simulink model "hybrid-grid-agc-simulink"  (R2025a)
settings: Solver=VariableStepAuto  StartTime=0.0  StopTime=4  RelTol=1e-3
libraries: spsSeriesRLCBranchLib x2, spsThreePhaseVIMeasurementLib x2, spsControlledVoltageSourceLib x1, spsGroundLib x1, spsPLL3phLib x1, eePwmGeneratorTwoLevel x1, spsSimplifiedSynchronousMachineSIUnitsLib x1, spsSteamTurbineandGovernorLib x1, spsThreePhaseParallelRLCLoadLib x1, spsThreePhaseSourceLib x1, spsUniversalBridgeLib x1, spsVoltageMeasurementLib x1
settings Model: Creator=saranshagrawal  LastModifiedBy=saranshagrawal

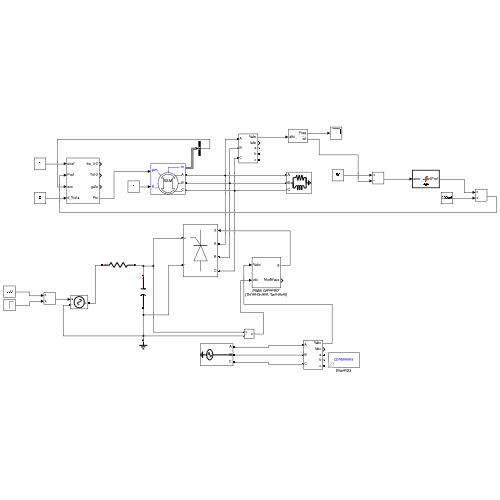
[thumbnail: Simulink's stored preview of the top-level diagram]
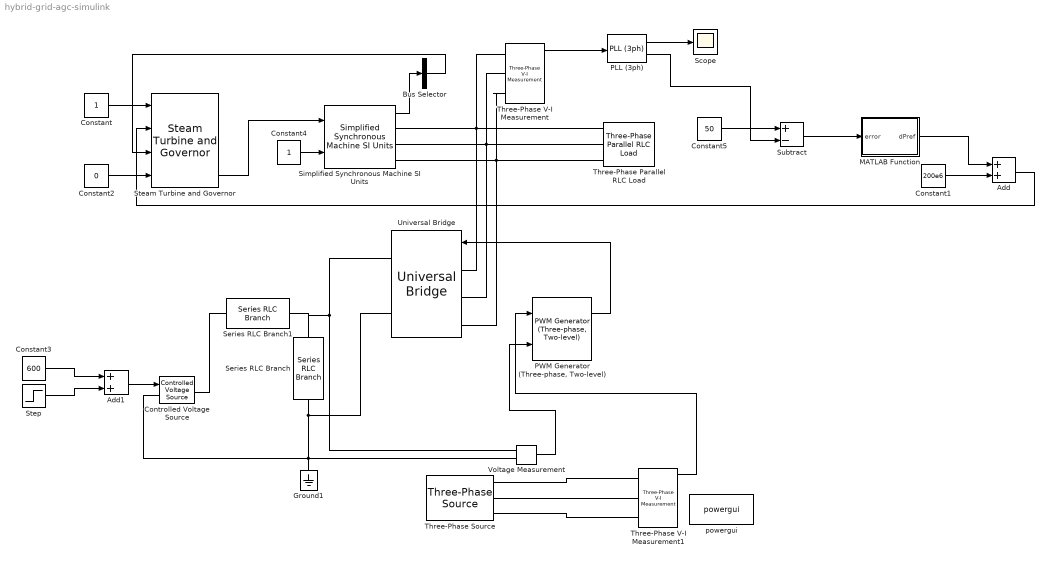
== system hybrid-grid-agc-simulink ==
  Add : Sum
  Add1 : Sum
  Bus Selector : BusSelector  OutputSignals=Rotor speed wm (rad/s)  OutputAsBus=on
  Constant : Constant
  Constant1 : Constant  Value=200e6
  Constant2 : Constant  Value=0
  Constant3 : Constant  Value=600
  Constant4 : Constant
  Constant5 : Constant  Value=50
  Controlled Voltage Source : spsControlledVoltageSourceLib/Controlled Voltage Source  Initialize=on  Source_Type=AC  Amplitude=0  Phase=0  Frequency=0  Measurements=None
  Ground1 : spsGroundLib/Ground  LConnTagsString=a
  MATLAB Function : MATLAB Function  TreatAsAtomicUnit=on
  PLL (3ph) : spsPLL3phLib/PLL (3ph)  Fmin=45  Par_Init=[0, 50]  ParK=[180, 3200, 1]  TcD=1e-4  MaxRateChangeFreq=12  FilterCutOffFreq=25  Ts=0  AGC=on
  "PWM Generator (Three-phase, Two-level)" : eePwmGeneratorTwoLevel/PWM Generator (Three-phase, Two-level)  PWMMode=Continuous PWM (CPWM)  CPWMMode=SPWM: sinusoidal PWM  DPWMMode=60 DPWM: 60 degree discontinuous PWM  fsw=1e3  Ts=5e-5
      settings: LibrarySourceBlock=|
      | ee_sl_lib/Pulse Width
      | Modulation/PWM Generator
      | (Three-phase, Two-level)
  Scope : Scope
      settings: ActiveDisplayYMinimum=49.969171432706709  ActiveDisplayYMaximum=50.039963228671333
  Series RLC Branch : spsSeriesRLCBranchLib/Series RLC Branch  LConnTagsString=__new0  RConnTagsString=__new0  BranchType=C  Resistance=1  Inductance=1e-3  SetiL0=off  InitialCurrent=0  Capacitance=1000e-6  Setx0=off  InitialVoltage=0  Measurements=None
  Series RLC Branch1 : spsSeriesRLCBranchLib/Series RLC Branch  LConnTagsString=__new0  RConnTagsString=__new0  BranchType=R  Resistance=1  Inductance=1e-3  SetiL0=off  InitialCurrent=0  Capacitance=1e-6  Setx0=off  InitialVoltage=0  Measurements=None
  Simplified Synchronous Machine SI Units : spsSimplifiedSynchronousMachineSIUnitsLib/Simplified Synchronous Machine SI Units  ConnectionType=3-wire Y  MechanicalLoad=Mechanical power Pm  MeasurementBus=off  NominalParameters=[187e6 13800 50]  Mechanical=[3.895e6 0 20]  InternalRL="[0.0204  0.8104e-3]"  InitialConditions="[ 0,0   0,0,0   0,0,0 ]"  IterativeDiscreteModel=Trapezoidal non iterative  TsBlock=-1  TsPowergui=0  LoadFlowParameters=[1,0,0,0,0]  Units=1  BusType=PV  Pref=0  Qref=0  Qmin=-inf  Qmax=+inf  PLF=0  QLF=0
      settings: LibrarySourceBlock=|
      | sps_lib/Electrical Machines/Simplified Synchronous
      | Machine SI Units
  Steam Turbine and Governor : spsSteamTurbineandGovernorLib/Steam Turbine and Governor  gentype=Tandem-compound (multi-mass)  reg1="[ 1  0.05    0 ]"  reg2="[ 0.001  0.15 ]"  reg3="[ -0.1  0.1  0  4.496]"  N=3000  turb1="[ 0  10   3.3   0.5   ]"  turb2="[ 0.5   0.5   0  0 ]"  HA="[  1.5498   0.24894  0  0 ]"  KA="[  83.47  42.702  0  0 ]"  DA=[2.4832 0.4 0 0]  ini1=250.35/555  ini2=[0 -120]
      settings: LibrarySourceBlock=|
      | sps_lib/Electrical Machines/Synchronous Machine Control/Steam Turbine
      | and Governor
  Step : Step  Time=2  After=500  SampleTime=0
  Subtract : Sum  Inputs=+-
  Three-Phase Parallel RLC Load : spsThreePhaseParallelRLCLoadLib/Three-Phase Parallel RLC Load  LConnTagsString=A|B|C  Configuration=Y (grounded)  NominalVoltage=1000  Vabc=[1e3 1e3 1e3]  Vabcp=[1e3 1e3 1e3]  NominalFrequency=50  UnbalancedPower=off  ActivePower=40e6  InductivePower=10e6  CapacitivePower=0  Pabc=[10e3 9e3 11e3]  QLabc=[100 90 110]  QCabc=[100 90 110]  Pabcp=[10e3 9e3 11e3]  QLabcp=[100 90 110]  QCabcp=[100 90 110]  Measurements=None  LoadType=constant Z
  Three-Phase V-I Measurement : spsThreePhaseVIMeasurementLib/Three-Phase V-I Measurement  VoltageMeasurement=phase-to-ground  SetLabelV=off  LabelV=Vabc  Vpu=off  VpuLL=off  CurrentMeasurement=yes  SetLabelI=off  LabelI=Iabc  Ipu=off  Pbase=100e6  Vbase=500e3  OutputType=Complex  PhasorSimulation=off  PSBequivalent=0
  Three-Phase V-I Measurement1 : spsThreePhaseVIMeasurementLib/Three-Phase V-I Measurement  VoltageMeasurement=phase-to-ground  SetLabelV=off  LabelV=Vabc  Vpu=off  VpuLL=off  CurrentMeasurement=yes  SetLabelI=off  LabelI=Iabc  Ipu=off  Pbase=100e6  Vbase=500e3  OutputType=Complex  PhasorSimulation=off  PSBequivalent=0
  Three-Phase Source : spsThreePhaseSourceLib/Three-Phase Source  InternalConnection=Yg  VoltagePhases=off  Voltage=1  PhaseAngle=0  Voltage_phases=[25e3 25e3 25e3]/sqrt(3)  PhaseAngles_phases=[0 -120 +120]  Frequency=50  NonIdealSource=on  SpecifyImpedance=off  Resistance=0  Inductance=0  ShortCircuitLevel=100e6  BaseVoltage=1  XRratio=7  BusType=swing  Pref=10e3  Qref=0  Prefabc=[10e3, 10e3, 10e3]  Qrefabc=[0, 0, 0]  Qmin=-inf  Qmax=inf
  Universal Bridge : spsUniversalBridgeLib/Universal Bridge  Arms=3  SnubberResistance=1e5  SnubberCapacitance=inf  Device=Thyristors  Ron=1e-3  Lon=0  ForwardVoltages="[  0  0  ]"  ForwardVoltage=0  GTOparameters=[ 10e-6 , 20e-6 ]  IGBTparameters=[ 1e-6 , 2e-6 ]  Measurements=None  Measurements_2=None  converterType=Rectifier
  Voltage Measurement : spsVoltageMeasurementLib/Voltage Measurement  PhasorSimulation=off  OutputType=Complex  PSBequivalent=0
  powergui : sps_lib/powergui  Priority=1  SimulationMode=Continuous  SampleTime=50e-6  frequency=60  Iterations=50  frequencyindice=50  Pbase=100e6  ErrMax=1e-4  UnitsV=kV  UnitsW=MW  buscounter=0  FunctionMessages=off  echomessages=off  EnableUseOfTLC=off  CurrentSourceSwitches=off  DisableSnubberDevices=off  DisableRonSwitches=off  DisableVfSwitches=off  DisplayEquations=off  AutomaticDiscreteSolvers=off  SolverType=Tustin/Backward Euler (TBE)  Interpol=off  ExternalGateDelay=off  methode=off  Ts=100  x0status=blocks  SPID=on  SwTol=0  HookPort=off  NonlinearTolerance=1e-4  nMaxIteration=100  ContinueOnMaxIteration=off  RestoreLinks=warning  ResistiveCurrentMeasurement=off  Frange=[0:2:500]  Ylog=off  Xlog=on  ShowGrid=off  save=off  variable=ZData  structure=0  ZoomFFT=off  StartTime=0.0  cycles=1  DisplayStyle=1  fundamental=60  FreqAxis=off  MaxFrequency=1000  frequencyindicesteady=1  RmsSteady=1  display=off
  wires:
  Steam Turbine and Governor/4 -> Simplified Synchronous Machine SI Units/1
  Constant/1 -> Steam Turbine and Governor/1
  Constant2/1 -> Steam Turbine and Governor/4
  Constant4/1 -> Simplified Synchronous Machine SI Units/2
  Three-Phase V-I Measurement/1 -> PLL (3ph)/1
  PLL (3ph)/1 -> Scope/1
  Constant5/1 -> Subtract/1
  PLL (3ph)/2 -> Subtract/2
  Subtract/1 -> MATLAB Function/1(error)
  MATLAB Function/1(dPref) -> Add/1
  Constant1/1 -> Add/2
  Add/1 -> Steam Turbine and Governor/2
  Simplified Synchronous Machine SI Units/1 -> Bus Selector/1
  Bus Selector/1 -> Steam Turbine and Governor/3
  Three-Phase V-I Measurement1/1 -> "PWM Generator (Three-phase, Two-level)"/1
  "PWM Generator (Three-phase, Two-level)"/1 -> Universal Bridge/1
  Voltage Measurement/1 -> "PWM Generator (Three-phase, Two-level)"/2
  Constant3/1 -> Add1/1
  Step/1 -> Add1/2
  Add1/1 -> Controlled Voltage Source/1
  connections:
  Universal Bridge/RConn1 -- Series RLC Branch/LConn1 -- Series RLC Branch1/RConn1 -- Voltage Measurement/LConn1
  Ground1/LConn1 -- Universal Bridge/RConn2 -- Series RLC Branch/RConn1 -- Controlled Voltage Source/LConn1 -- Voltage Measurement/LConn2
  Three-Phase Source/RConn1 -- Three-Phase V-I Measurement1/LConn1
  Three-Phase Source/RConn2 -- Three-Phase V-I Measurement1/LConn2
  Three-Phase Source/RConn3 -- Three-Phase V-I Measurement1/LConn3
  Universal Bridge/LConn1 -- Three-Phase V-I Measurement/LConn1 -- Three-Phase Parallel RLC Load/LConn1 -- Simplified Synchronous Machine SI Units/RConn1
  Universal Bridge/LConn2 -- Three-Phase Parallel RLC Load/LConn2 -- Three-Phase V-I Measurement/LConn2 -- Simplified Synchronous Machine SI Units/RConn2
  Simplified Synchronous Machine SI Units/RConn3 -- Universal Bridge/LConn3 -- Three-Phase Parallel RLC Load/LConn3 -- Three-Phase V-I Measurement/LConn3
  Controlled Voltage Source/RConn1 -- Series RLC Branch1/LConn1

== matlab function hybrid-grid-agc-simulink/MATLAB Function ==
  settings: updateMethod=DISCRETE
  data: error input; dPref output
function dPref = agc(error)

persistent integral
if isempty(integral)
    integral = 0;
end

% Controller gains (tune later)
Kp = 5e4;
Ki = 1e3;

% Simulation time step (VERY IMPORTANT)
Ts = 1e-4;   % match your simulation step (or approx)

% Integrator
integral = integral + error * Ts;

% PI controller output (this is ΔPref, not total Pref)
dPref = Kp*error + Ki*integral;

% Limit output (to avoid instability)
dPref = max(min(dPref, 50e6), -50e6);

end
